simulink model "DCmotor"  (R2020b)
settings: Solver=VariableStepAuto  StartTime=0.0  StopTime=10.0  RelTol=1e-3
settings Model: DataDictionary=DataDictionary.sldd  Creator=abhin  LastModifiedBy=abhin

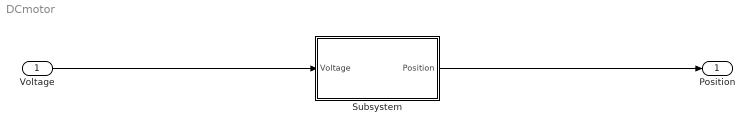
== system DCmotor ==
  Voltage : Inport
  Subsystem : Subsystem
  Position : Outport
  wires:
  Voltage/1 -> Subsystem/1(Voltage)
  Subsystem/1(Position) -> Position/1

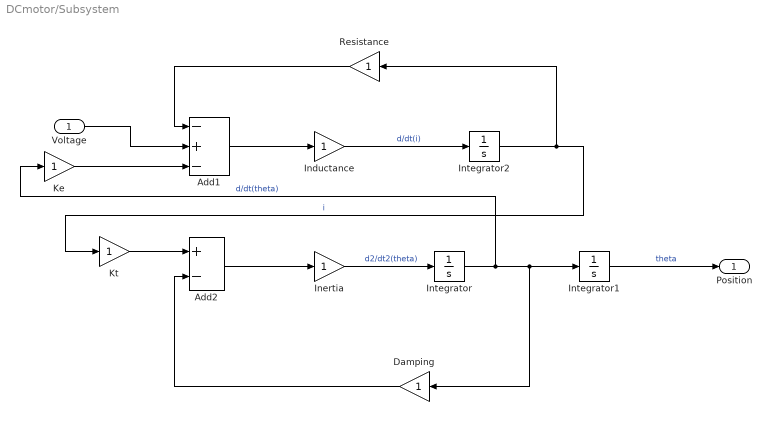
== system DCmotor/Subsystem ==
  Voltage : Inport
  Add1 : Sum  Inputs=-+-
  Add2 : Sum  Inputs=+-
  Damping : Gain
  Inductance : Gain
  Inertia : Gain
  Integrator : Integrator
  Integrator1 : Integrator
  Integrator2 : Integrator
  Ke : Gain
  Kt : Gain
  Resistance : Gain
  Position : Outport
  wires:
  Integrator1/1 -> Position/1  "theta"
  Inductance/1 -> Integrator2/1  "d/dt(i)"
  Integrator2/1 -> Resistance/1, Kt/1  "i"
  Resistance/1 -> Add1/1
  Integrator/1 -> Ke/1, Damping/1, Integrator1/1  "d/dt(theta)"
  Inertia/1 -> Integrator/1  "d2/dt2(theta)"
  Add2/1 -> Inertia/1
  Voltage/1 -> Add1/2
  Add1/1 -> Inductance/1
  Kt/1 -> Add2/1
  Damping/1 -> Add2/2
  Ke/1 -> Add1/3
